simulink library "LumAerospaceBlockset_Payloads"  (R2021a)
settings: Solver=ode45  StartTime=0.0  StopTime=10.0  RelTol=1e-3  EnableMultiTasking=on
undefined symbols (not defined in the file): payload
libraries: LumAerospaceBlockset_Utilities x3, $bdroot x2
settings Model: Creator=Christopher  LastModifiedBy=chris
settings SolverCC: AlgebraicLoopSolver=TrustRegion
settings DataIOCC: LimitDataPoints=on  SaveFormat=Array  ReturnWorkspaceOutputs=off
settings OptimizationCC: LifeSpan=inf
settings DebuggingCC: SolverPrmCheckMsg=warning  SFUnexpectedBacktrackingDiag=warning  SFNoUnconditionalDefaultTransitionDiag=warning  SFExecutionAtInitializationDiag=none  SFMachineParentedDataDiag=warning  ArithmeticOperatorsInVariantConditions=warning
settings HardwareCC: ProdBitPerPointer=32  ProdBitPerSizeT=32  ProdBitPerPtrDiffT=32  ProdLargestAtomicFloat=None  ProdIntDivRoundTo=Undefined  ProdEndianess=Unspecified  ProdWordSize=32  ProdHWDeviceType=32-bit Generic
settings ModelReferenceCC: PropagateSignalLabelsOutOfModel=off
settings SFSimCC: SimUseLocalCustomCode=off  CustomCodeUndefinedFunction=UseInterfaceOnly
settings RTWCC: RTWUseLocalCustomCode=off
settings CodeAppCC: StateflowObjectComments=on
settings GRTTargetCC: TargetLangStandard=C89/C90 (ANSI)
settings ConfigComp: CovMetricSettings=dw  CovSaveCumulativeToWorkspaceVar=on  CovSaveSingleToWorkspaceVar=on  CovExternalEMLEnable=off  CovSFcnEnable=off

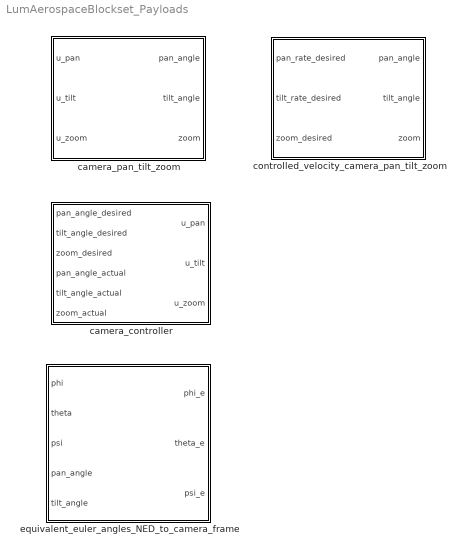
== system LumAerospaceBlockset_Payloads ==
  camera_controller : Subsystem
      mask help:
      | Implement a simple, inner loop controller for the camera
      |
      | INPUT:  -pan_angle_desired: desired pan angle (rad)
      |         -tilt_angle_desired: desired tilt angle (rad)
      |         -zoom_desired: desired zoom factor
      |         -pan_angle_actual: actual pan angle (rad)
      |         -tilt_angle_actual: actual tilt angle (rad)
      |         -zoom_actual: actual zoom factor
      |
      | OUTPUT: -u_pan: control signal in range [-1,1] (1 = increase pan angle at max rate, -1 = decrease...)
      |         -u_tilt: control signal in range [-1,1] (1 = increase tilt angle at max rate, -1 = decrease...)
      |         -u_zoom: control signal in range [-1,1] (1 = increase zoom factor at max rate, -1 = decrease...)
      |
      | VALIDATION: -none
  camera_pan_tilt_zoom : Subsystem  mask{initial_pan=payload.camera.initial_pan_angle, max_pan_rate=payload.camera.pan_rate, max_pan=payload.camera.pan_angle_max, min_pan=payload.camera.pan_angle_min, initial_tilt=payload.camera.initial_tilt_angle, max_tilt_rate=payload.camera.tilt_rate, max_tilt=payload.camera.tilt_angle_max, min_tilt=payload.camera.tilt_angle_min, initial_zoom=payload.camera.initial_zoom, max_zoom_rate=payload.camera.zoom_rate, max_zoom=payload.camera.zoom_max, min_zoom=payload.camera.zoom_min}
      mask prompts: initial_pan "Initial pan angle (rad)"; max_pan_rate "Maximum pan rate (rad/s)"; max_pan "Maximum pan angle (rad)"; min_pan "Minimum pan angle (rad)"; initial_tilt "Initial tilt angle (rad)"; max_tilt_rate "Maximum tilt rate (rad/s)"; max_tilt "Maximum tilt angle (rad)"; min_tilt "Minimum tilt angle (rad)"; initial_zoom "Initial zoom (unitless)"; max_zoom_rate "Maximum zoom rate (units/s)"; max_zoom "Maximum zoom (unitless)"; min_zoom "Minimum zoom (unitless)"
      mask help:
      | Model a camera with a pan angle, tilt angle, and zoom factor.
      |
      | INPUT:  -u_pan:  value in range [-1,1] (1 = increase pan angle at maximum pan rate, -1 = decrease...)
      |         -u_tilt: value in range [-1,1] (1 = increase tilt angle at maximum pan rate, -1 = decrease...)
      |         -u_zoom: value in range [-1,1] (1 = increase zoom factor at maximum zoom rate, -1 = decrease...)
      |
      | OUTPUT: -pan_angle: pan angle of camera (rad)
      |         -tilt_angle: tilt angle of camera (rad)
      |         -zoom: zoom factor of camera
      |
      | VALIDATION: -none
  controlled_velocity_camera_pan_tilt_zoom : Subsystem  mask{initial_pan=payload.camera.initial_pan_angle, max_pan_rate=payload.camera.pan_rate, max_pan=payload.camera.pan_angle_max, min_pan=payload.camera.pan_angle_min, initial_tilt=payload.camera.initial_tilt_angle, max_tilt_rate=payload.camera.tilt_rate, max_tilt=payload.camera.tilt_angle_max, min_tilt=payload.camera.tilt_angle_min, initial_zoom=payload.camera.initial_zoom, max_zoom_rate=payload.camera.zoom_rate, max_zoom=payload.camera.zoom_max, min_zoom=payload.camera.zoom_min}
      mask prompts: initial_pan "Initial pan angle (rad)"; max_pan_rate "Maximum pan rate (rad/s)"; max_pan "Maximum pan angle (rad)"; min_pan "Minimum pan angle (rad)"; initial_tilt "Initial tilt angle (rad)"; max_tilt_rate "Maximum tilt rate (rad/s)"; max_tilt "Maximum tilt angle (rad)"; min_tilt "Minimum tilt angle (rad)"; initial_zoom "Initial zoom (unitless)"; max_zoom_rate "Maximum zoom rate (units/s)"; max_zoom "Maximum zoom (unitless)"; min_zoom "Minimum zoom (unitless)"
      mask help:
      | Model a camera with a pan angle, tilt angle, and zoom factor.
      |
      | The camera is controlled in the sense that the user can specify desired rates and zoom factor and the camera will attempt to track these signals.
      |
      | INPUT:  -pan_rate_desired:  desired pan anglular rate (rad/s)
      |         -tilt_rate_desired: desired tilt angular rate (rad/s)
      |         -zoom_desired: desired zoom factor
      |
      | OUTPUT: -pan_angle: pan angle of camera (rad)
      |         -tilt_angle: tilt angle of camera (rad)
      |         -zoom: zoom factor of camera
      |
      | VALIDATION: -unit test
  equivalent_euler_angles_NED_to_camera_frame : Subsystem
      mask help:
      | This block works for a camera which is in line with the body frame but can be panned (yawed) and tilted (pitched).
      |
      | A positive pan is about the body z axis and goes from the body frame to the 3 frame.
      |
      | A positive tilt is about the 3 frame y axis and goes from the 3 frame to the camera frame.
      |
      | If the aircraft is at the attitude specified by the euler angles phi, theta, psi and the camera orientation is specified by the pan_angle and tilt_angle, this block will compute the equivalent 3 Euler rotations which go from the NED frame to the camera frame.
      |
      | INPUT:  -phi:   bank angle of aircraft (rad)
      |         -theta: pitch angle of aircraft (rad)
      |         -psi:   yaw angle of aircraft (rad)
      |         -pan_angle: pan angle of camera (rad)
      |         -tilt_angle:    tilt angle of camera (rad)
      |
      | OUTPUT: -phi_e: equivalent roll euler angle to go from NED to camera frame (rad)
      |         -theta_e: equivalent pitch euler angle to go from NED to camera frame (rad)
      |         -psi_e:  equivalent yaw euler angle to go from NED to camera frame (rad)

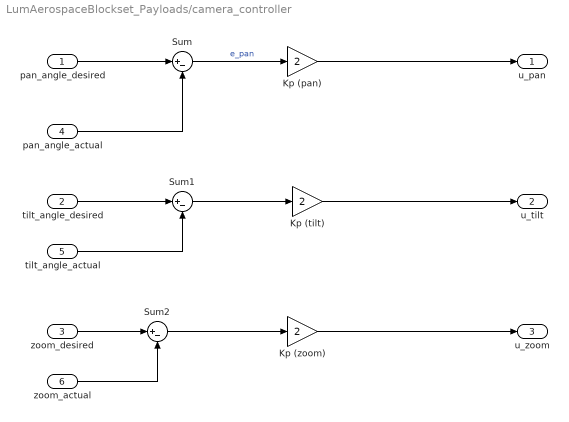
== system LumAerospaceBlockset_Payloads/camera_controller ==
  pan_angle_desired : Inport
  tilt_angle_desired : Inport  Port=2
  zoom_desired : Inport  Port=3
  pan_angle_actual : Inport  Port=4
  tilt_angle_actual : Inport  Port=5
  zoom_actual : Inport  Port=6
  Kp (pan) : Gain  Gain=2
  Kp (tilt) : Gain  Gain=2
  Kp (zoom) : Gain  Gain=2
  Sum : Sum  Inputs=|+-
  Sum1 : Sum  Inputs=|+-
  Sum2 : Sum  Inputs=|+-
  u_pan : Outport
  u_tilt : Outport  Port=2
  u_zoom : Outport  Port=3
  wires:
  pan_angle_desired/1 -> Sum/1
  pan_angle_actual/1 -> Sum/2
  Kp (pan)/1 -> u_pan/1
  Sum/1 -> Kp (pan)/1  "e_pan"
  tilt_angle_desired/1 -> Sum1/1
  tilt_angle_actual/1 -> Sum1/2
  Sum1/1 -> Kp (tilt)/1
  Kp (tilt)/1 -> u_tilt/1
  zoom_desired/1 -> Sum2/1
  zoom_actual/1 -> Sum2/2
  Sum2/1 -> Kp (zoom)/1
  Kp (zoom)/1 -> u_zoom/1

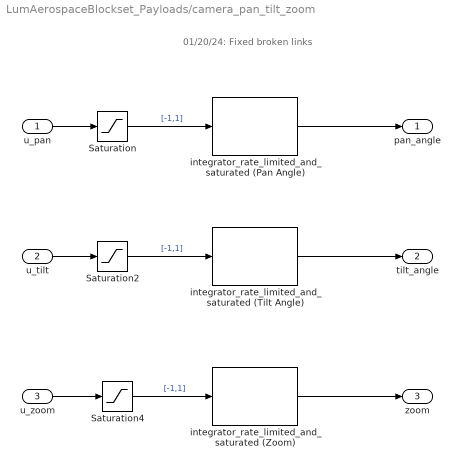
== system LumAerospaceBlockset_Payloads/camera_pan_tilt_zoom ==
  note: 01/20/24: Fixed broken links
  u_pan : Inport
  u_tilt : Inport  Port=2
  u_zoom : Inport  Port=3
  Saturation : Saturate  UpperLimit=1  LowerLimit=-1
  Saturation2 : Saturate  UpperLimit=1  LowerLimit=-1
  Saturation4 : Saturate  UpperLimit=1  LowerLimit=-1
  integrator_rate_limited_and_saturated (Pan Angle) : LumAerospaceBlockset_Utilities/integrator_rate_limited_and_saturated  x0=initial_pan  rate_gain=max_pan_rate  x_max=max_pan  x_min=min_pan
  integrator_rate_limited_and_saturated (Tilt Angle) : LumAerospaceBlockset_Utilities/integrator_rate_limited_and_saturated  x0=initial_tilt  rate_gain=max_tilt_rate  x_max=max_tilt  x_min=min_tilt
  integrator_rate_limited_and_saturated (Zoom) : LumAerospaceBlockset_Utilities/integrator_rate_limited_and_saturated  x0=initial_zoom  rate_gain=max_zoom_rate  x_max=max_zoom  x_min=min_zoom
  pan_angle : Outport
  tilt_angle : Outport  Port=2
  zoom : Outport  Port=3
  wires:
  integrator_rate_limited_and_saturated (Pan Angle)/1 -> pan_angle/1
  integrator_rate_limited_and_saturated (Tilt Angle)/1 -> tilt_angle/1
  u_pan/1 -> Saturation/1
  u_tilt/1 -> Saturation2/1
  Saturation/1 -> integrator_rate_limited_and_saturated (Pan Angle)/1  "[-1,1]"
  Saturation2/1 -> integrator_rate_limited_and_saturated (Tilt Angle)/1  "[-1,1]"
  Saturation4/1 -> integrator_rate_limited_and_saturated (Zoom)/1  "[-1,1]"
  u_zoom/1 -> Saturation4/1
  integrator_rate_limited_and_saturated (Zoom)/1 -> zoom/1

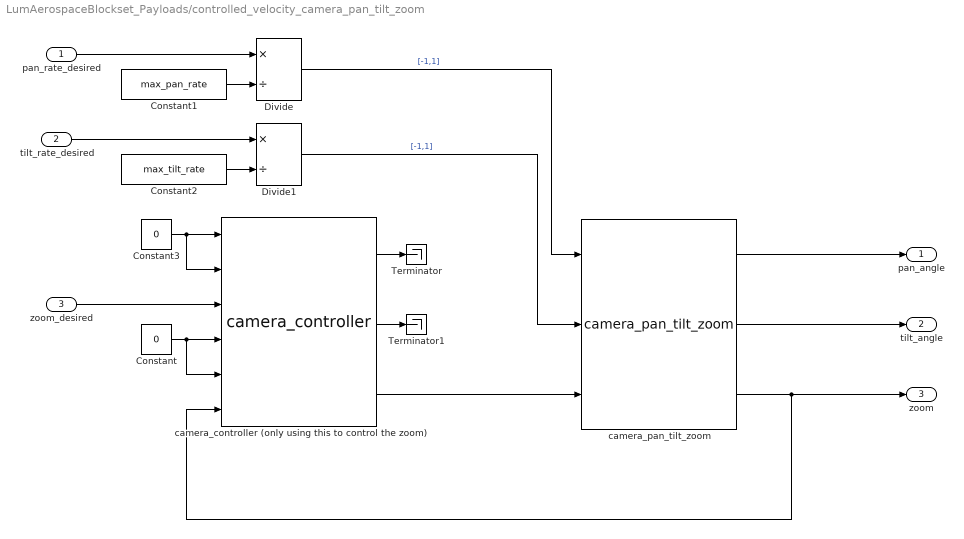
== system LumAerospaceBlockset_Payloads/controlled_velocity_camera_pan_tilt_zoom ==
  pan_rate_desired : Inport
  tilt_rate_desired : Inport  Port=2
  zoom_desired : Inport  Port=3
  Constant : Constant  Value=0
  Constant1 : Constant  Value=max_pan_rate
  Constant2 : Constant  Value=max_tilt_rate
  Constant3 : Constant  Value=0
  Divide : Product  Inputs=*/
  Divide1 : Product  Inputs=*/
  Terminator : Terminator
  Terminator1 : Terminator
  camera_controller (only using this to control the zoom) : $bdroot/camera_controller
  camera_pan_tilt_zoom : $bdroot/camera_pan_tilt_zoom  initial_pan=initial_pan  max_pan_rate=max_pan_rate  max_pan=max_pan  min_pan=min_pan  initial_tilt=initial_tilt  max_tilt_rate=max_tilt_rate  max_tilt=max_tilt  min_tilt=min_tilt  initial_zoom=initial_zoom  max_zoom_rate=max_zoom_rate  max_zoom=max_zoom  min_zoom=min_zoom
  pan_angle : Outport
  tilt_angle : Outport  Port=2
  zoom : Outport  Port=3
  wires:
  zoom_desired/1 -> camera_controller (only using this to control the zoom)/3
  tilt_rate_desired/1 -> Divide1/1
  pan_rate_desired/1 -> Divide/1
  camera_controller (only using this to control the zoom)/3 -> camera_pan_tilt_zoom/3
  camera_pan_tilt_zoom/3 -> camera_controller (only using this to control the zoom)/6, zoom/1
  camera_pan_tilt_zoom/2 -> tilt_angle/1
  camera_pan_tilt_zoom/1 -> pan_angle/1
  Constant/1 -> camera_controller (only using this to control the zoom)/5, camera_controller (only using this to control the zoom)/4
  camera_controller (only using this to control the zoom)/1 -> Terminator/1
  camera_controller (only using this to control the zoom)/2 -> Terminator1/1
  Constant1/1 -> Divide/2
  Divide/1 -> camera_pan_tilt_zoom/1  "[-1,1]"
  Constant2/1 -> Divide1/2
  Divide1/1 -> camera_pan_tilt_zoom/2  "[-1,1]"
  Constant3/1 -> camera_controller (only using this to control the zoom)/2, camera_controller (only using this to control the zoom)/1

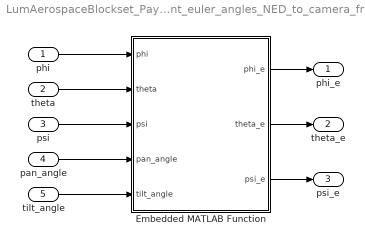
== system LumAerospaceBlockset_Payloads/equivalent_euler_angles_NED_to_camera_frame ==
  phi : Inport
  theta : Inport  Port=2
  psi : Inport  Port=3
  pan_angle : Inport  Port=4
  tilt_angle : Inport  Port=5
  Embedded MATLAB Function : MATLAB Function  TreatAsAtomicUnit=on
  phi_e : Outport
  theta_e : Outport  Port=2
  psi_e : Outport  Port=3
  wires:
  Embedded MATLAB Function/1(phi_e) -> phi_e/1
  Embedded MATLAB Function/2(theta_e) -> theta_e/1
  Embedded MATLAB Function/3(psi_e) -> psi_e/1
  phi/1 -> Embedded MATLAB Function/1(phi)
  theta/1 -> Embedded MATLAB Function/2(theta)
  psi/1 -> Embedded MATLAB Function/3(psi)
  pan_angle/1 -> Embedded MATLAB Function/4(pan_angle)
  tilt_angle/1 -> Embedded MATLAB Function/5(tilt_angle)

== matlab function LumAerospaceBlockset_Payloads/equivalent_euler_angles_NED_to_camera_frame/Embedded MATLAB Function ==
  data: phi input; phi_e output; theta input; psi input; pan_angle input; tilt_angle input; theta_e output; psi_e output
function [phi_e, theta_e, psi_e] = fcn(phi, theta, psi, pan_angle, tilt_angle)

%Generate various rotation matrices to go from NED frame to body frame
C_1v = [cos(psi) sin(psi) 0
    -sin(psi) cos(psi) 0
    0 0 1];

C_21 = [cos(theta) 0 -sin(theta);
    0 1 0;
    sin(theta) 0 cos(theta)];

C_b2 = [1 0 0;
    0 cos(phi) sin(phi);
    0 -sin(phi) cos(phi)];

%Now what are the rotation matrices to go from both to camera frame
psi_c = pan_angle;
theta_c = tilt_angle;

C_3b = [cos(psi_c) sin(psi_c) 0;
    -sin(psi_c) cos(psi_c) 0
    0 0 1];

C_c3 = [cos(theta_c) 0 -sin(theta_c);
    0 1 0;
    sin(theta_c) 0 cos(theta_c)];

%Now generate the direction cosines matrix to go from NED frame to camera
%frame
C_cv = C_c3*C_3b*C_b2*C_21*C_1v;

%We can now extract the equivalent 3 euler angles which would go from the
%NED frame to the camera frame
theta_e = -asin(C_cv(1,3));
phi_e = atan2(C_cv(2,3), C_cv(3,3));
psi_e = atan2(C_cv(1,2), C_cv(1,1));
